simulink model "cds_simulink_file"  (R2020b)
settings: Solver=ode5  StartTime=0.0  StopTime=5  FixedStep=Ts  RelTol=1e-3
values from neighbouring files (symbols this model uses):
  D = (m2+mp/3)*9.81*[1;1;1;0]    [cds_main_bsmc_sigma.m]    (also in cds_model.m = ((m2+mp/3)*9.81)*[1;1;1;0]+external_force; cds_plant_sigma.m = ((m2+mp/3)*9.81+ef)*[1;1;1;0]; myIneqConFunction.m = ((m2+mp/3)*9.81)*[1;1;1;0]+external_force)
  PredictionHorizon = 5    [modelLyna_sm_withnoise (run first).m]
  Ts = 0.05    [modelLyna_sm_withnoise (run first).m]    (also in myIneqConFunction.m = data.Ts)
  u0 = [0;0;0;0]    [modelLyna_sm_withnoise (run first).m]
  x0 = [0*ones(3993,1); 0*ones(7,1)]    [cds_fuzzy_bsmc_sigma.m]    (also in cds_fuzzy_l_sigma.m; cds_main_bsmc_sigma.m = []; cds_plant_sigma.m = [0.45 0.7 0.5 0 0 0 0 0]; cds_setpoint_mpc.m = [])
undefined symbols (not defined in the file or in its folder): ref
libraries: mpclib x1
settings Model: Creator=Dell Precision  LastModifiedBy=Dell Precision
settings SFSimCC: CustomCodeUndefinedFunction=UseInterfaceOnly

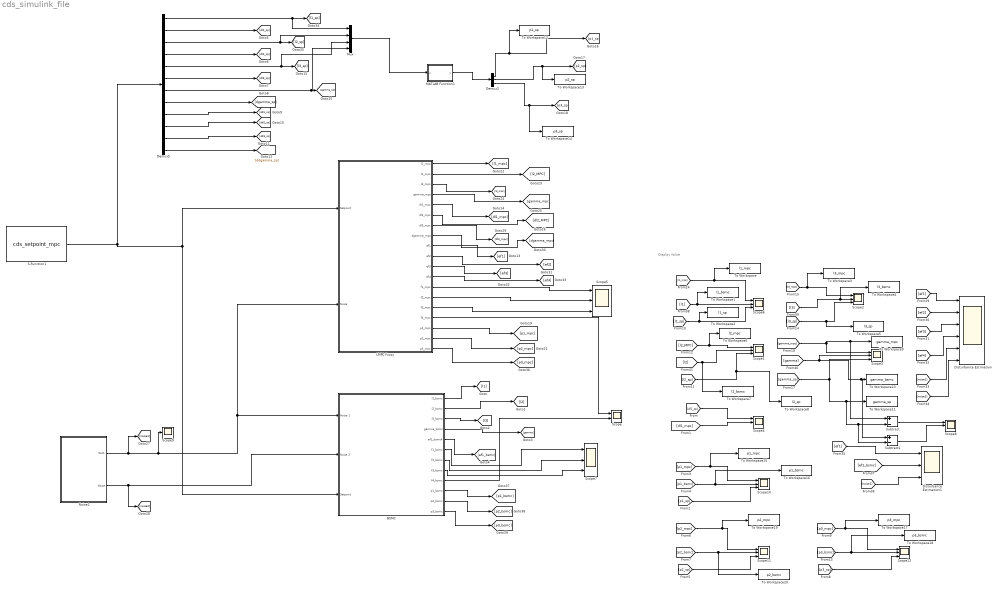
== system cds_simulink_file ==
  note: Display Value
  BSMC : Subsystem
  Demux2 : Demux  Outputs=3
  Demux5 : Demux  Outputs=12
  Disturbance Estimation : Scope  NumInputPorts=6
  Disturbance Estimation1 : Scope  NumInputPorts=3
  LMPC Fuzzy : Subsystem
  MATLAB Function1 : MATLAB Function  TreatAsAtomicUnit=on
  Mux : Mux
  Noise2 : Subsystem
  S-Function1 : S-Function  FunctionName=cds_setpoint_mpc  SFunctionDeploymentMode=off  EnableBusSupport=off
  Scope : Scope  NumInputPorts=2
  Scope{1..8,10..12} (11 alike) : Scope  NumInputPorts=3
  Scope9 : Scope
  Subtract : Sum  Inputs=+-
  Subtract1 : Sum  Inputs=+-
  To Workspace : ToWorkspace  VariableName=l1_mpc  SaveFormat=Timeseries  SampleTime=-1
  To Workspace1 : ToWorkspace  VariableName=l1_bsmc  SaveFormat=Timeseries  SampleTime=-1
  To Workspace10 : ToWorkspace  VariableName=gamma_bsmc  SaveFormat=Timeseries  SampleTime=-1
  To Workspace11 : ToWorkspace  VariableName=gamma_sp  SaveFormat=Timeseries  SampleTime=-1
  To Workspace12 : ToWorkspace  VariableName=p1_sp  SaveFormat=Timeseries  SampleTime=-1
  To Workspace13 : ToWorkspace  VariableName=p2_sp  SaveFormat=Timeseries  SampleTime=-1
  To Workspace14 : ToWorkspace  VariableName=p3_sp  SaveFormat=Timeseries  SampleTime=-1
  To Workspace15 : ToWorkspace  VariableName=p1_mpc  SaveFormat=Timeseries  SampleTime=-1
  To Workspace16 : ToWorkspace  VariableName=p1_bsmc  SaveFormat=Timeseries  SampleTime=-1
  To Workspace17 : ToWorkspace  VariableName=p3_mpc  SaveFormat=Timeseries  SampleTime=-1
  To Workspace18 : ToWorkspace  VariableName=p3_bsmc  SaveFormat=Timeseries  SampleTime=-1
  To Workspace19 : ToWorkspace  VariableName=p2_mpc  SaveFormat=Timeseries  SampleTime=-1
  To Workspace2 : ToWorkspace  VariableName=l1_sp  SaveFormat=Timeseries  SampleTime=-1
  To Workspace20 : ToWorkspace  VariableName=p2_bsmc  SaveFormat=Timeseries  SampleTime=-1
  To Workspace3 : ToWorkspace  VariableName=l3_mpc  SaveFormat=Timeseries  SampleTime=-1
  To Workspace4 : ToWorkspace  VariableName=l3_bsmc  SaveFormat=Timeseries  SampleTime=-1
  To Workspace5 : ToWorkspace  VariableName=l3_sp  SaveFormat=Timeseries  SampleTime=-1
  To Workspace6 : ToWorkspace  VariableName=l2_mpc  SaveFormat=Timeseries  SampleTime=-1
  To Workspace7 : ToWorkspace  VariableName=l2_bsmc  SaveFormat=Timeseries  SampleTime=-1
  To Workspace8 : ToWorkspace  VariableName=l2_sp  SaveFormat=Timeseries  SampleTime=-1
  To Workspace9 : ToWorkspace  VariableName=gamma_mpc  SaveFormat=Timeseries  SampleTime=-1
  wires:
  [l1_mpc] -> To Workspace/1, Scope6/1
  Noise2/2(Noise) -> BSMC/2(Noise 2), [noise2]
  [l3_sp] -> To Workspace5/1, Scope2/3
  [noise2] -> Disturbance Estimation/6
  [noise1] -> Disturbance Estimation/5
  [gamma_mpc] -> Subtract/1, To Workspace9/1, Scope3/1
  [l1_sp] -> To Workspace2/1, Scope6/3
  [l2_sp] -> To Workspace8/1, Scope1/3
  [ef2] -> Disturbance Estimation/2
  [ef1] -> Disturbance Estimation/1
  [ef3] -> Disturbance Estimation/3
  [l3_mpc] -> To Workspace3/1, Scope2/1
  [ef4] -> Disturbance Estimation/4
  Noise2/1(Out1) -> Scope9/1, LMPC Fuzzy/2(Noise), BSMC/1(Noise 1), [noise1]
  [gamma_sp] -> Subtract1/2, Subtract/2, To Workspace11/1, Scope3/3
  [ef1] -> Disturbance Estimation1/1
  [noise1] -> Disturbance Estimation1/3
  [ef1_bsmc] -> Disturbance Estimation1/2
  [l1] -> To Workspace1/1, Scope6/2
  [l3] -> To Workspace4/1, Scope2/2
  [gamma] -> Scope3/2, Subtract1/1, To Workspace10/1
  [l2] -> To Workspace7/1, Scope1/2
  LMPC Fuzzy/1(l1_mpc) -> [l1_mpc]
  LMPC Fuzzy/2(l2_mpc) -> [l2_MPC]
  LMPC Fuzzy/3(l3_mpc) -> [l3_mpc]
  LMPC Fuzzy/4(gamma_mpc) -> [gamma_mpc]
  LMPC Fuzzy/5(dl1_mpc) -> [dl1_mpc]
  LMPC Fuzzy/6(dl2_mpc) -> [dl2_MPC]
  LMPC Fuzzy/7(dl3_mpc) -> [dl3_mpc]
  LMPC Fuzzy/8(dgamma_mpc) -> [dgamma_mpc]
  LMPC Fuzzy/9(ef1) -> [ef1]
  LMPC Fuzzy/10(ef2) -> [ef2]
  LMPC Fuzzy/11(ef3) -> [ef3]
  LMPC Fuzzy/12(ef4) -> [ef4]
  [dl1_sp] -> Scope4/1
  [dl1_mpc] -> Scope4/2
  BSMC/1(l1_bsmc) -> [l1]
  BSMC/2(l2_bsmc) -> [l2]
  BSMC/3(l3_bsmc) -> [l3]
  BSMC/4(gamma_bsmc) -> [gamma]
  BSMC/5(ef1_bsmc4) -> [ef1_bsmc]
  Demux5/12 -> [ddgamma_sp]
  Demux5/8 -> [dgamma_sp]
  Demux5/9 -> [ddl1_sp]
  Demux5/5 -> Mux/3, [l3_sp]
  Demux5/4 -> [dl2_sp]
  S-Function1/1 -> Demux5/1, BSMC/3(Setpoint), LMPC Fuzzy/1(Setpoint)
  Demux5/2 -> [dl1_sp]
  Demux5/7 -> Mux/4, [gamma_sp]
  Demux5/10 -> [ddl2_sp]
  Demux5/3 -> Mux/2, [l2_sp]
  Demux5/1 -> Mux/1, [l1_sp]
  Demux5/11 -> [ddl3_sp]
  Demux5/6 -> [dl3_sp]
  [l2_MPC] -> To Workspace6/1, Scope1/1
  LMPC Fuzzy/13(f1_mpc) -> Scope5/1
  LMPC Fuzzy/14(f2_mpc) -> Scope5/2
  LMPC Fuzzy/15(f3_mpc) -> Scope5/3
  BSMC/6(f1_bsmc) -> Scope7/1
  BSMC/7(f2_bsmc) -> Scope7/2
  BSMC/8(f3_bsmc) -> Scope7/3
  LMPC Fuzzy/16(f4_mpc) -> Scope/1
  BSMC/9(f4_bsmc) -> Scope/2
  Subtract/1 -> Scope8/1
  Subtract1/1 -> Scope8/2
  Demux2/1 -> To Workspace12/1, [p1_sp]
  MATLAB Function1/1(y) -> Demux2/1
  Demux2/2 -> To Workspace13/1, [p2_sp]
  Demux2/3 -> To Workspace14/1, [p3_sp]
  Mux/1 -> MATLAB Function1/1(u)
  LMPC Fuzzy/17(p1_mpc) -> [p1_mpc]
  LMPC Fuzzy/18(p2_mpc) -> [p2_mpc]
  LMPC Fuzzy/19(p3_mpc) -> [p3_mpc]
  BSMC/10(p1_bsmc) -> [p1_bsmc]
  BSMC/11(p2_bsmc) -> [p2_bsmc]
  BSMC/12(p3_bsmc) -> [p3_bsmc]
  [p1_sp] -> Scope10/3
  [p2_mpc] -> To Workspace19/1, Scope11/1
  [p2_sp] -> Scope11/3
  [p2_bsmc] -> To Workspace20/1, Scope11/2
  [p3_bsmc] -> To Workspace18/1, Scope12/2
  [p3_sp] -> Scope12/3
  [p3_mpc] -> To Workspace17/1, Scope12/1
  [p1_mpc] -> To Workspace15/1, Scope10/1
  [p1_bsmc] -> To Workspace16/1, Scope10/2

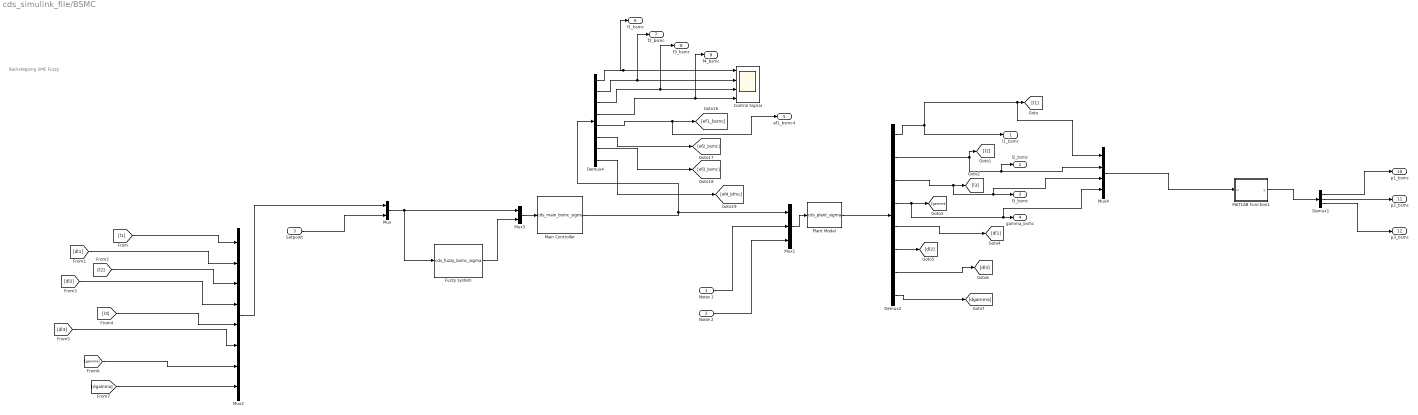
== system cds_simulink_file/BSMC ==
  note: Backstepping SMC Fuzzy
  Noise 1 : Inport
  Noise 2 : Inport  Port=2
  Setpoint : Inport  Port=3
  Control Signal : Scope  NumInputPorts=4
  Demux1 : Demux  Outputs=3
  Demux2 : Demux  Outputs=8
  Demux4 : Demux  Outputs=8
  Fuzzy system : S-Function  FunctionName=cds_fuzzy_bsmc_sigma  SFunctionDeploymentMode=off  EnableBusSupport=off
  MATLAB Function1 : MATLAB Function  TreatAsAtomicUnit=on
  Main Controller : S-Function  FunctionName=cds_main_bsmc_sigma  SFunctionDeploymentMode=off  EnableBusSupport=off
  Mux : Mux  Inputs=2
  Mux1 : Mux  Inputs=3
  Mux2 : Mux  Inputs=8
  Mux3 : Mux  Inputs=2
  Mux4 : Mux
  Plant Model : S-Function  FunctionName=cds_plant_sigma  SFunctionDeploymentMode=off  EnableBusSupport=off
  l1_bsmc : Outport
  l2_bsmc : Outport  Port=2
  l3_bsmc : Outport  Port=3
  gamma_bsmc : Outport  Port=4
  ef1_bsmc4 : Outport  Port=5
  f1_bsmc : Outport  Port=6
  f2_bsmc : Outport  Port=7
  f3_bsmc : Outport  Port=8
  f4_bsmc : Outport  Port=9
  p1_bsmc : Outport  Port=10
  p2_bsmc : Outport  Port=11
  p3_bsmc : Outport  Port=12
  wires:
  Demux4/4 -> f4_bsmc/1, Control Signal/4
  Mux/1 -> Mux3/1, Fuzzy system/1
  Fuzzy system/1 -> Mux3/2
  Demux2/6 -> [dl2]
  Main Controller/1 -> Demux4/1, Mux1/1
  Demux2/1 -> l1_bsmc/1, Mux4/1, [l1]
  [dl2] -> Mux2/4
  [gamma] -> Mux2/7
  Noise 2/1 -> Mux1/3
  [l3] -> Mux2/5
  [l2] -> Mux2/3
  Noise 1/1 -> Mux1/2
  [dgamma] -> Mux2/8
  [dl3] -> Mux2/6
  Demux4/6 -> [ef2_bsmc]
  Plant Model/1 -> Demux2/1
  Setpoint/1 -> Mux/2
  Demux4/8 -> [ef4_bfmc]
  Demux2/3 -> Mux4/3, l3_bsmc/1, [l3]
  Demux2/8 -> [dgamma]
  Demux4/5 -> ef1_bsmc4/1, [ef1_bsmc]
  Demux4/1 -> f1_bsmc/1, Control Signal/1
  Mux2/1 -> Mux/1
  Demux4/7 -> [ef3_bsmc]
  [dl1] -> Mux2/2
  [l1] -> Mux2/1
  Demux2/5 -> [dl1]
  Demux4/3 -> f3_bsmc/1, Control Signal/3
  Demux2/2 -> Mux4/2, l2_bsmc/1, [l2]
  Mux1/1 -> Plant Model/1
  Demux2/4 -> Mux4/4, gamma_bsmc/1, [gamma]
  Demux2/7 -> [dl3]
  Mux3/1 -> Main Controller/1
  Demux4/2 -> f2_bsmc/1, Control Signal/2
  Demux1/1 -> p1_bsmc/1
  MATLAB Function1/1(y) -> Demux1/1
  Demux1/2 -> p2_bsmc/1
  Demux1/3 -> p3_bsmc/1
  Mux4/1 -> MATLAB Function1/1(u)

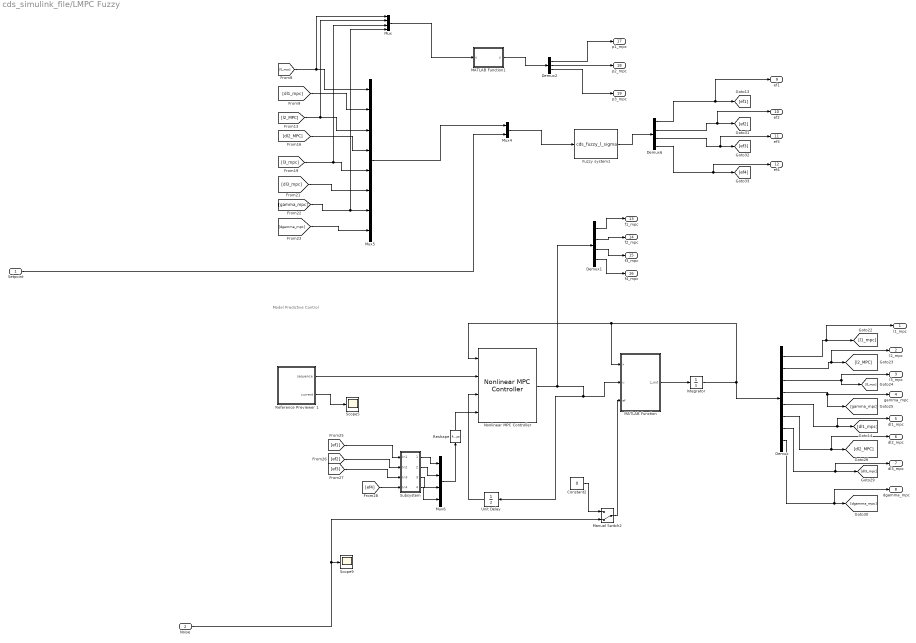
== system cds_simulink_file/LMPC Fuzzy ==
  note: Model Predictive Control
  Setpoint : Inport
  Noise : Inport  Port=2
  Constant2 : Constant  Value=0
  Demux : Demux  Outputs=8
  Demux1 : Demux
  Demux2 : Demux  Outputs=3
  Demux6 : Demux
  Fuzzy system1 : S-Function  FunctionName=cds_fuzzy_l_sigma  SFunctionDeploymentMode=off  EnableBusSupport=off
  Integrator : Integrator  InitialCondition=x0
  MATLAB Function : MATLAB Function  TreatAsAtomicUnit=on
  MATLAB Function1 : MATLAB Function  TreatAsAtomicUnit=on
  Manual Switch2 : ManualSwitch  CurrentSetting=0
  Mux : Mux
  Mux4 : Mux  Inputs=2
  Mux5 : Mux  Inputs=8
  Mux6 : Mux
  Nonlinear MPC Controller : mpclib/Nonlinear MPC Controller  SCDEnableBlockLinearizationSpecification=on  nlmpcobj=nlobj  UseObjectTs=on  UseMEX=off  md_enabled=on  mvtarget_enabled=off  param_enabled=off  cost_enabled=off  mvseq_enabled=off  stateseq_enabled=off  ovseq_enabled=off  slack_enabled=off  status_enabled=off  ov_min=off  ov_max=off  mv_min=off  mv_max=off  mvrate_min=off  mvrate_max=off  state_min=off  state_max=off  ov_weight=off  mv_weight=off  mvrate_weight=off  ecr_weight=off  nlp_initialize=off
  Reference Previewer 1 : Subsystem  mask{signal=ref, ts=Ts, steps=PredictionHorizon}
      mask prompts: signal "Signal name"; ts "Sampling time"; steps "Number of previewing steps"
      mask init:
      | ts = evalin('base',get_param(gcbh,'ts'));
      | signal = evalin('base',get_param(gcbh,'signal'));
      | steps = evalin('base',get_param(gcbh,'steps'));
      | data = mpc_previewer_maskinit(signal,ts);
      mask Display:
      | fprintf('Future\nsample\nextractor');
      | port_label('output', 1, 'seq')
      | port_label('output', 2, '@t')
  Reshape : Reshape  OutputDimensionality=Row vector (2-D)
  Scope5 : Scope
  Scope9 : Scope
  Subsystem : Subsystem
  Unit Delay : UnitDelay  InitialCondition=u0  SampleTime=-1  HasFrameUpgradeWarning=on
  l1_mpc : Outport
  l2_mpc : Outport  Port=2
  l3_mpc : Outport  Port=3
  gamma_mpc : Outport  Port=4
  dl1_mpc : Outport  Port=5
  dl2_mpc : Outport  Port=6
  dl3_mpc : Outport  Port=7
  dgamma_mpc : Outport  Port=8
  ef1 : Outport  Port=9
  ef2 : Outport  Port=10
  ef3 : Outport  Port=11
  ef4 : Outport  Port=12
  f1_mpc : Outport  Port=13
  f2_mpc : Outport  Port=14
  f3_mpc : Outport  Port=15
  f4_mpc : Outport  Port=16
  p1_mpc : Outport  Port=17
  p2_mpc : Outport  Port=18
  p3_mpc : Outport  Port=19
  wires:
  Manual Switch2/1 -> MATLAB Function/3(ef)
  Integrator/1 -> MATLAB Function/1(x), Nonlinear MPC Controller/1, Demux/1
  Demux/6 -> dl2_mpc/1, [dl2_MPC]
  Demux6/3 -> ef3/1, [ef3]
  [dl1_mpc] -> Mux5/2
  Demux/2 -> l2_mpc/1, [l2_MPC]
  MATLAB Function/1(z_out) -> Integrator/1
  Unit Delay/1 -> Nonlinear MPC Controller/3
  Demux6/4 -> ef4/1, [ef4]
  Demux6/2 -> ef2/1, [ef2]
  Reference Previewer 1/2(current) -> Scope5/1
  [dl2_MPC] -> Mux5/4
  [dl3_mpc] -> Mux5/6
  Mux6/1 -> Reshape/1
  Demux/5 -> dl1_mpc/1, [dl1_mpc]
  Noise/1 -> Manual Switch2/2, Scope9/1
  [ef4] -> Subsystem/4(In4)
  Demux/8 -> dgamma_mpc/1, [dgamma_mpc]
  Subsystem/1(Out1) -> Mux6/1
  Subsystem/3(Out3) -> Mux6/3
  [ef3] -> Subsystem/3(In3)
  Setpoint/1 -> Mux4/2
  [gamma_mpc] -> Mux/4, Mux5/7
  Fuzzy system1/1 -> Demux6/1
  Mux5/1 -> Mux4/1
  Reshape/1 -> Nonlinear MPC Controller/4
  Nonlinear MPC Controller/1 -> Demux1/1, MATLAB Function/2(u), Unit Delay/1
  Constant2/1 -> Manual Switch2/1
  Reference Previewer 1/1(sequence) -> Nonlinear MPC Controller/2
  Subsystem/4(Out4) -> Mux6/4
  Demux/3 -> l3_mpc/1, [l3_mpc]
  Subsystem/2(Out2) -> Mux6/2
  [l2_MPC] -> Mux/2, Mux5/3
  Demux/4 -> [gamma_mpc], gamma_mpc/1
  Demux/7 -> dl3_mpc/1, [dl3_mpc]
  [ef1] -> Subsystem/1(In1)
  [l1_mpc] -> Mux/1, Mux5/1
  Demux/1 -> l1_mpc/1, [l1_mpc]
  Mux4/1 -> Fuzzy system1/1
  [l3_mpc] -> Mux/3, Mux5/5
  [dgamma_mpc] -> Mux5/8
  [ef2] -> Subsystem/2(In2)
  Demux6/1 -> ef1/1, [ef1]
  Demux1/1 -> f1_mpc/1
  Demux1/2 -> f2_mpc/1
  Demux1/3 -> f3_mpc/1
  Demux1/4 -> f4_mpc/1
  Mux/1 -> MATLAB Function1/1(u)
  MATLAB Function1/1(y) -> Demux2/1
  Demux2/1 -> p1_mpc/1
  Demux2/2 -> p2_mpc/1
  Demux2/3 -> p3_mpc/1

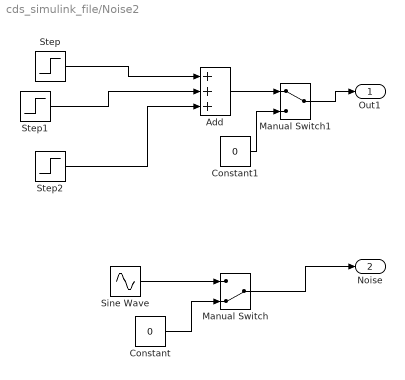
== system cds_simulink_file/Noise2 ==
  Add : Sum  Inputs=+++
  Constant : Constant  Value=0  SampleTime=-1
  Constant1 : Constant  Value=0  SampleTime=-1
  Manual Switch : ManualSwitch  CurrentSetting=0
  Manual Switch1 : ManualSwitch
  Sine Wave : Sin  Amplitude=25  Bias=25  Frequency=4  Phase=pi/2  SampleTime=0
  Step : Step  After=50  SampleTime=0
  Step1 : Step  Time=2  After=-80  SampleTime=0
  Step2 : Step  Time=4  After=60  SampleTime=0
  Out1 : Outport
  Noise : Outport  Port=2
  wires:
  Step/1 -> Add/1
  Step2/1 -> Add/3
  Step1/1 -> Add/2
  Sine Wave/1 -> Manual Switch/1
  Constant/1 -> Manual Switch/2
  Manual Switch/1 -> Noise/1
  Add/1 -> Manual Switch1/1
  Manual Switch1/1 -> Out1/1
  Constant1/1 -> Manual Switch1/2

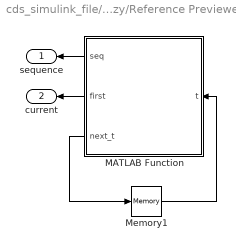
== system cds_simulink_file/LMPC Fuzzy/Reference Previewer 1 ==
  MATLAB Function : MATLAB Function  TreatAsAtomicUnit=on
  Memory1 : Memory  InheritSampleTime=on  LinearizeAsDelay=on
  sequence : Outport  VectorParamsAs1DForOutWhenUnconnected=off
  current : Outport  Port=2  VectorParamsAs1DForOutWhenUnconnected=off
  wires:
  MATLAB Function/1(seq) -> sequence/1
  MATLAB Function/2(first) -> current/1
  Memory1/1 -> MATLAB Function/1(t)
  MATLAB Function/3(next_t) -> Memory1/1

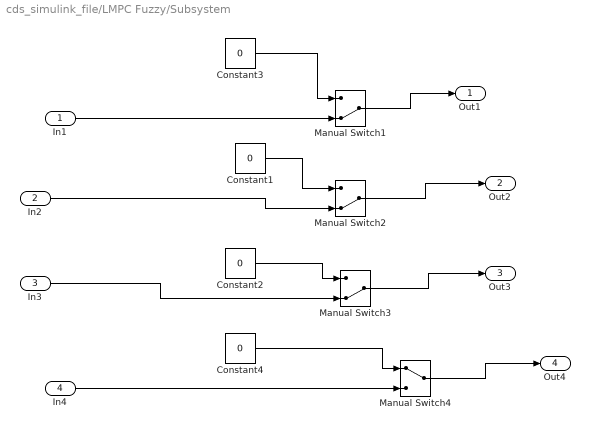
== system cds_simulink_file/LMPC Fuzzy/Subsystem ==
  In1 : Inport
  In2 : Inport  Port=2
  In3 : Inport  Port=3
  In4 : Inport  Port=4
  Constant{1..4} (4 alike) : Constant  Value=0
  Manual Switch1 : ManualSwitch  CurrentSetting=0
  Manual Switch2 : ManualSwitch  CurrentSetting=0
  Manual Switch3 : ManualSwitch  CurrentSetting=0
  Manual Switch4 : ManualSwitch
  Out1 : Outport
  Out2 : Outport  Port=2
  Out3 : Outport  Port=3
  Out4 : Outport  Port=4
  wires:
  Constant3/1 -> Manual Switch1/1
  Manual Switch1/1 -> Out1/1
  In1/1 -> Manual Switch1/2
  Manual Switch2/1 -> Out2/1
  Constant1/1 -> Manual Switch2/1
  Constant2/1 -> Manual Switch3/1
  Manual Switch3/1 -> Out3/1
  Manual Switch4/1 -> Out4/1
  Constant4/1 -> Manual Switch4/1
  In2/1 -> Manual Switch2/2
  In3/1 -> Manual Switch3/2
  In4/1 -> Manual Switch4/2

== matlab function cds_simulink_file/LMPC Fuzzy/MATLAB Function1 ==
  data: u input; y output
function y = cal_inv(u)

%% input

q = u(1:4);

l1 = q(1);
l2 = q(2);
l3 = q(3);
gamma = q(4);
a = 0.5;
az = 0.05;

A1 = [a*sin(pi/6) a*cos(pi/6) 0]';
A2 = [-a 0 0]';
A3 = [a*sin(pi/6) -a*cos(pi/6) 0]';


B1 = [a*sin(pi/6) a*cos(pi/6) 0]';
B2 = [-a 0 0]';
B3 = [a*sin(pi/6) -a*cos(pi/6) 0]';



X = [150;0;0];

for i = 1:100

    Pz = X(1);    
    alpha = X(2);
    beta = X(3);

Rp = [cos(beta)*cos(gamma) cos(gamma)*sin(alpha)*sin(beta)-cos(alpha)*sin(gamma) sin(alpha)*sin(gamma)+cos(alpha)*cos(gamma)*sin(beta);
      cos(beta)*sin(gamma) cos(alpha)*cos(gamma)+sin(alpha)*sin(beta)*sin(gamma) cos(alpha)*sin(beta)*sin(gamma)-cos(gamma)*sin(alpha);
      -sin(beta)                    cos(beta)*sin(alpha)                                        cos(alpha)*cos(beta)                   ];
Ra = [cos(gamma) -sin(gamma) 0;
      sin(gamma) cos(gamma)  0; 
           0         0       1];
       


Oa = [0 0 az]';
P  = [0 0 Pz]';

f1 = (Rp*B1 + P - Ra*A1 - Oa)'*(Rp*B1 + P - Ra*A1 - Oa) - l1^2  ;
f2 = (Rp*B2 + P - Ra*A2 - Oa)'*(Rp*B2 + P - Ra*A2 - Oa) - l2^2  ;
f3 = (Rp*B3 + P - Ra*A3 - Oa)'*(Rp*B3 + P - Ra*A3 - Oa) - l3^2  ;

df1z = Pz - az + conj(Pz) - conj(az) - (a*sin(conj(beta)))/2 - (conj(a)*sin(beta))/2 + (3^(1/2)*conj(a)*cos(beta)*sin(alpha))/2 + (3^(1/2)*a*cos(conj(beta))*sin(conj(alpha)))/2;
 
 
df1_alpha = (3^(1/2)*a*(cos(conj(gamma))*sin(conj(alpha)) - cos(conj(alpha))*sin(conj(beta))*sin(conj(gamma)))*((conj(a)*sin(gamma))/2 + (3^(1/2)*conj(a)*cos(gamma))/2 - (conj(a)*cos(beta)*cos(gamma))/2 - (3^(1/2)*conj(a)*(cos(alpha)*cos(gamma) + sin(alpha)*sin(beta)*sin(gamma)))/2))/2 - (3^(1/2)*a*(sin(conj(alpha))*sin(conj(gamma)) + cos(conj(alpha))*cos(conj(gamma))*sin(conj(beta)))*((conj(a)*cos(gamma))/2 - (3^(1/2)*conj(a)*sin(gamma))/2 - (conj(a)*cos(beta)*cos(gamma))/2 + (3^(1/2)*conj(a)*(cos(alpha)*sin(gamma) - cos(gamma)*sin(alpha)*sin(beta)))/2))/2 - (3^(1/2)*conj(a)*(sin(alpha)*sin(gamma) + cos(alpha)*cos(gamma)*sin(beta))*((a*cos(conj(gamma)))/2 - (a*cos(conj(beta))*cos(conj(gamma)))/2 + (3^(1/2)*a*(cos(conj(alpha))*sin(conj(gamma)) - cos(conj(gamma))*sin(conj(alpha))*sin(conj(beta))))/2 - (3^(1/2)*a*sin(conj(gamma)))/2))/2 + (3^(1/2)*conj(a)*(cos(gamma)*sin(alpha) - cos(alpha)*sin(beta)*sin(gamma))*((a*sin(conj(gamma)))/2 - (a*cos(conj(beta))*cos(conj(gamma)))/2 - (3^(1/2)*a*(cos(conj(alpha))*cos(conj(gamma)) + sin(conj(alpha))*sin(conj(beta))*sin(conj(gamma))))/2 + (3^(1/2)*a*cos(conj(gamma)))/2))/2 + (3^(1/2)*a*cos(conj(alpha))*cos(conj(beta))*(conj(Pz) - conj(az) - (conj(a)*sin(beta))/2 + (3^(1/2)*conj(a)*cos(beta)*sin(alpha))/2))/2 + (3^(1/2)*conj(a)*cos(alpha)*cos(beta)*(Pz - az - (a*sin(conj(beta)))/2 + (3^(1/2)*a*cos(conj(beta))*sin(conj(alpha)))/2))/2;
 
 
df1_beta = ((conj(a)*cos(gamma)*sin(beta))/2 - (3^(1/2)*conj(a)*cos(beta)*cos(gamma)*sin(alpha))/2)*((a*cos(conj(gamma)))/2 - (a*cos(conj(beta))*cos(conj(gamma)))/2 + (3^(1/2)*a*(cos(conj(alpha))*sin(conj(gamma)) - cos(conj(gamma))*sin(conj(alpha))*sin(conj(beta))))/2 - (3^(1/2)*a*sin(conj(gamma)))/2) + ((conj(a)*cos(gamma)*sin(beta))/2 - (3^(1/2)*conj(a)*cos(beta)*sin(alpha)*sin(gamma))/2)*((a*sin(conj(gamma)))/2 - (a*cos(conj(beta))*cos(conj(gamma)))/2 - (3^(1/2)*a*(cos(conj(alpha))*cos(conj(gamma)) + sin(conj(alpha))*sin(conj(beta))*sin(conj(gamma))))/2 + (3^(1/2)*a*cos(conj(gamma)))/2) - ((a*cos(conj(beta)))/2 + (3^(1/2)*a*sin(conj(alpha))*sin(conj(beta)))/2)*(conj(Pz) - conj(az) - (conj(a)*sin(beta))/2 + (3^(1/2)*conj(a)*cos(beta)*sin(alpha))/2) + ((a*cos(conj(gamma))*sin(conj(beta)))/2 - (3^(1/2)*a*cos(conj(beta))*cos(conj(gamma))*sin(conj(alpha)))/2)*((conj(a)*cos(gamma))/2 - (3^(1/2)*conj(a)*sin(gamma))/2 - (conj(a)*cos(beta)*cos(gamma))/2 + (3^(1/2)*conj(a)*(cos(alpha)*sin(gamma) - cos(gamma)*sin(alpha)*sin(beta)))/2) + ((a*cos(conj(gamma))*sin(conj(beta)))/2 - (3^(1/2)*a*cos(conj(beta))*sin(conj(alpha))*sin(conj(gamma)))/2)*((conj(a)*sin(gamma))/2 + (3^(1/2)*conj(a)*cos(gamma))/2 - (conj(a)*cos(beta)*cos(gamma))/2 - (3^(1/2)*conj(a)*(cos(alpha)*cos(gamma) + sin(alpha)*sin(beta)*sin(gamma)))/2) - ((conj(a)*cos(beta))/2 + (3^(1/2)*conj(a)*sin(alpha)*sin(beta))/2)*(Pz - az - (a*sin(conj(beta)))/2 + (3^(1/2)*a*cos(conj(beta))*sin(conj(alpha)))/2);
 
 
df2z = Pz - az + conj(Pz) - conj(az) + a*sin(conj(beta)) + conj(a)*sin(beta);
 
 
df2_alpha = 0;
 
 
df2_beta = a*cos(conj(beta))*(conj(Pz) - conj(az) + conj(a)*sin(beta)) + conj(a)*cos(beta)*(Pz - az + a*sin(conj(beta))) + a*cos(conj(gamma))*sin(conj(beta))*(conj(a)*cos(gamma) - conj(a)*cos(beta)*cos(gamma)) + conj(a)*cos(gamma)*sin(beta)*(a*cos(conj(gamma)) - a*cos(conj(beta))*cos(conj(gamma))) + a*cos(conj(gamma))*sin(conj(beta))*(conj(a)*sin(gamma) - conj(a)*cos(beta)*cos(gamma)) + conj(a)*cos(gamma)*sin(beta)*(a*sin(conj(gamma)) - a*cos(conj(beta))*cos(conj(gamma)));
 
 
df3z = Pz - az + conj(Pz) - conj(az) - (a*sin(conj(beta)))/2 - (conj(a)*sin(beta))/2 - (3^(1/2)*conj(a)*cos(beta)*sin(alpha))/2 - (3^(1/2)*a*cos(conj(beta))*sin(conj(alpha)))/2;
 
 
df3_alpha = (3^(1/2)*a*(sin(conj(alpha))*sin(conj(gamma)) + cos(conj(alpha))*cos(conj(gamma))*sin(conj(beta)))*((conj(a)*cos(gamma))/2 + (3^(1/2)*conj(a)*sin(gamma))/2 - (conj(a)*cos(beta)*cos(gamma))/2 - (3^(1/2)*conj(a)*(cos(alpha)*sin(gamma) - cos(gamma)*sin(alpha)*sin(beta)))/2))/2 - (3^(1/2)*a*(cos(conj(gamma))*sin(conj(alpha)) - cos(conj(alpha))*sin(conj(beta))*sin(conj(gamma)))*((conj(a)*sin(gamma))/2 - (3^(1/2)*conj(a)*cos(gamma))/2 - (conj(a)*cos(beta)*cos(gamma))/2 + (3^(1/2)*conj(a)*(cos(alpha)*cos(gamma) + sin(alpha)*sin(beta)*sin(gamma)))/2))/2 + (3^(1/2)*conj(a)*(sin(alpha)*sin(gamma) + cos(alpha)*cos(gamma)*sin(beta))*((a*cos(conj(gamma)))/2 - (a*cos(conj(beta))*cos(conj(gamma)))/2 - (3^(1/2)*a*(cos(conj(alpha))*sin(conj(gamma)) - cos(conj(gamma))*sin(conj(alpha))*sin(conj(beta))))/2 + (3^(1/2)*a*sin(conj(gamma)))/2))/2 - (3^(1/2)*conj(a)*(cos(gamma)*sin(alpha) - cos(alpha)*sin(beta)*sin(gamma))*((a*sin(conj(gamma)))/2 - (a*cos(conj(beta))*cos(conj(gamma)))/2 + (3^(1/2)*a*(cos(conj(alpha))*cos(conj(gamma)) + sin(conj(alpha))*sin(conj(beta))*sin(conj(gamma))))/2 - (3^(1/2)*a*cos(conj(gamma)))/2))/2 + (3^(1/2)*a*cos(conj(alpha))*cos(conj(beta))*(conj(az) - conj(Pz) + (conj(a)*sin(beta))/2 + (3^(1/2)*conj(a)*cos(beta)*sin(alpha))/2))/2 + (3^(1/2)*conj(a)*cos(alpha)*cos(beta)*(az - Pz + (a*sin(conj(beta)))/2 + (3^(1/2)*a*cos(conj(beta))*sin(conj(alpha)))/2))/2;
 
 
df3_beta = ((conj(a)*cos(gamma)*sin(beta))/2 + (3^(1/2)*conj(a)*cos(beta)*cos(gamma)*sin(alpha))/2)*((a*cos(conj(gamma)))/2 - (a*cos(conj(beta))*cos(conj(gamma)))/2 - (3^(1/2)*a*(cos(conj(alpha))*sin(conj(gamma)) - cos(conj(gamma))*sin(conj(alpha))*sin(conj(beta))))/2 + (3^(1/2)*a*sin(conj(gamma)))/2) + ((conj(a)*cos(gamma)*sin(beta))/2 + (3^(1/2)*conj(a)*cos(beta)*sin(alpha)*sin(gamma))/2)*((a*sin(conj(gamma)))/2 - (a*cos(conj(beta))*cos(conj(gamma)))/2 + (3^(1/2)*a*(cos(conj(alpha))*cos(conj(gamma)) + sin(conj(alpha))*sin(conj(beta))*sin(conj(gamma))))/2 - (3^(1/2)*a*cos(conj(gamma)))/2) + ((a*cos(conj(beta)))/2 - (3^(1/2)*a*sin(conj(alpha))*sin(conj(beta)))/2)*(conj(az) - conj(Pz) + (conj(a)*sin(beta))/2 + (3^(1/2)*conj(a)*cos(beta)*sin(alpha))/2) + ((a*cos(conj(gamma))*sin(conj(beta)))/2 + (3^(1/2)*a*cos(conj(beta))*cos(conj(gamma))*sin(conj(alpha)))/2)*((conj(a)*cos(gamma))/2 + (3^(1/2)*conj(a)*sin(gamma))/2 - (conj(a)*cos(beta)*cos(gamma))/2 - (3^(1/2)*conj(a)*(cos(alpha)*sin(gamma) - cos(gamma)*sin(alpha)*sin(beta)))/2) + ((a*cos(conj(gamma))*sin(conj(beta)))/2 + (3^(1/2)*a*cos(conj(beta))*sin(conj(alpha))*sin(conj(gamma)))/2)*((conj(a)*sin(gamma))/2 - (3^(1/2)*conj(a)*cos(gamma))/2 - (conj(a)*cos(beta)*cos(gamma))/2 + (3^(1/2)*conj(a)*(cos(alpha)*cos(gamma) + sin(alpha)*sin(beta)*sin(gamma)))/2) + ((conj(a)*cos(beta))/2 - (3^(1/2)*conj(a)*sin(alpha)*sin(beta))/2)*(az - Pz + (a*sin(conj(beta)))/2 + (3^(1/2)*a*cos(conj(beta))*sin(conj(alpha)))/2);

f = [f1 f2 f3]';

df = [df1z df1_alpha df1_beta;
      df2z df2_alpha df2_beta;   
      df3z df3_alpha df3_beta];

  
X = X - (df^(-1))*f;

end
 
X(1) = abs(X(1));
y = X;

end

== matlab function cds_simulink_file/LMPC Fuzzy/MATLAB Function ==
  data: x input; u input; z_out output; ef input
function z_out  = cds_model_sm(x,u, ef)

a = 0.5 ;                            % Some static parameters
mp = 15; m1 =0.5; m2 = 3; mdc =3; Ipy = 1; Ipx = 1; Igamma = 1;
m11 = m2 + mdc + mp/9 + Ipy/(4*a^2); m21 = mp/9;
m22 = m2+mdc+mp/9+ Ipx/(12*a^2); m33 = m2 +mdc +mp/9; m44 = Igamma;
M = [m11 m21 m21 0; m21 m22 m21 0; m21 m21 m33 0; 0 0 0 m44];
invM = inv(M);
c1 = 15*Ipy/(4*a^4) ; c2 = 5*Ipx/(12*a^4);
D = ((m2+mp/3)*9.81)*[1;1;1;0]+ ef*[1;1;1;0];

dl1 = x(5);
dl2 = x(6);
dl3 = x(7);
dgamma = x(8);
ddl1 =invM(1,1)*(u(1)-D(1)-c1*dl1*dl1)+invM(1,2)*(u(2) - D(2)-c2*dl2*dl2)+invM(1,3)*(u(3)-D(3))+invM(1,4)*(u(4)-D(4));
ddl2 =invM(2,1)*(u(1)-D(1)-c1*dl1*dl1)+invM(2,2)*(u(2) - D(2)-c2*dl2*dl2)+invM(2,3)*(u(3)-D(3))+invM(2,4)*(u(4)-D(4));
ddl3 =invM(3,1)*(u(1)-D(1)-c1*dl1*dl1)+invM(3,2)*(u(2) - D(2)-c2*dl2*dl2)+invM(3,3)*(u(3)-D(3))+invM(3,4)*(u(4)-D(4));
ddgamma =invM(4,4)*(u(4)-D(4));

z_out = [dl1;dl2;dl3;dgamma;ddl1;ddl2;ddl3;ddgamma];
end

== matlab function cds_simulink_file/LMPC Fuzzy/Reference Previewer 1/MATLAB Function ==
  settings: updateMethod=DISCRETE  sampleTime=ts
  data: data parameter; seq output; steps parameter; t input; first output; next_t output
function [seq,first,next_t] = fcn(data,steps,t)
%#codegen
[seq,first,next_t] = mpcblock_preview('ref',data,steps,t);

== matlab function cds_simulink_file/BSMC/MATLAB Function1 ==
  data: u input; y output
function y = cal_inv(u)

%% input

q = u(1:4);

l1 = q(1);
l2 = q(2);
l3 = q(3);
gamma = q(4);
a = 0.5;
az = 0.05;

A1 = [a*sin(pi/6) a*cos(pi/6) 0]';
A2 = [-a 0 0]';
A3 = [a*sin(pi/6) -a*cos(pi/6) 0]';


B1 = [a*sin(pi/6) a*cos(pi/6) 0]';
B2 = [-a 0 0]';
B3 = [a*sin(pi/6) -a*cos(pi/6) 0]';



X = [150;0;0];

for i = 1:100

    Pz = X(1);    
    alpha = X(2);
    beta = X(3);

Rp = [cos(beta)*cos(gamma) cos(gamma)*sin(alpha)*sin(beta)-cos(alpha)*sin(gamma) sin(alpha)*sin(gamma)+cos(alpha)*cos(gamma)*sin(beta);
      cos(beta)*sin(gamma) cos(alpha)*cos(gamma)+sin(alpha)*sin(beta)*sin(gamma) cos(alpha)*sin(beta)*sin(gamma)-cos(gamma)*sin(alpha);
      -sin(beta)                    cos(beta)*sin(alpha)                                        cos(alpha)*cos(beta)                   ];
Ra = [cos(gamma) -sin(gamma) 0;
      sin(gamma) cos(gamma)  0; 
           0         0       1];
       


Oa = [0 0 az]';
P  = [0 0 Pz]';

f1 = (Rp*B1 + P - Ra*A1 - Oa)'*(Rp*B1 + P - Ra*A1 - Oa) - l1^2  ;
f2 = (Rp*B2 + P - Ra*A2 - Oa)'*(Rp*B2 + P - Ra*A2 - Oa) - l2^2  ;
f3 = (Rp*B3 + P - Ra*A3 - Oa)'*(Rp*B3 + P - Ra*A3 - Oa) - l3^2  ;

df1z = Pz - az + conj(Pz) - conj(az) - (a*sin(conj(beta)))/2 - (conj(a)*sin(beta))/2 + (3^(1/2)*conj(a)*cos(beta)*sin(alpha))/2 + (3^(1/2)*a*cos(conj(beta))*sin(conj(alpha)))/2;
 
 
df1_alpha = (3^(1/2)*a*(cos(conj(gamma))*sin(conj(alpha)) - cos(conj(alpha))*sin(conj(beta))*sin(conj(gamma)))*((conj(a)*sin(gamma))/2 + (3^(1/2)*conj(a)*cos(gamma))/2 - (conj(a)*cos(beta)*cos(gamma))/2 - (3^(1/2)*conj(a)*(cos(alpha)*cos(gamma) + sin(alpha)*sin(beta)*sin(gamma)))/2))/2 - (3^(1/2)*a*(sin(conj(alpha))*sin(conj(gamma)) + cos(conj(alpha))*cos(conj(gamma))*sin(conj(beta)))*((conj(a)*cos(gamma))/2 - (3^(1/2)*conj(a)*sin(gamma))/2 - (conj(a)*cos(beta)*cos(gamma))/2 + (3^(1/2)*conj(a)*(cos(alpha)*sin(gamma) - cos(gamma)*sin(alpha)*sin(beta)))/2))/2 - (3^(1/2)*conj(a)*(sin(alpha)*sin(gamma) + cos(alpha)*cos(gamma)*sin(beta))*((a*cos(conj(gamma)))/2 - (a*cos(conj(beta))*cos(conj(gamma)))/2 + (3^(1/2)*a*(cos(conj(alpha))*sin(conj(gamma)) - cos(conj(gamma))*sin(conj(alpha))*sin(conj(beta))))/2 - (3^(1/2)*a*sin(conj(gamma)))/2))/2 + (3^(1/2)*conj(a)*(cos(gamma)*sin(alpha) - cos(alpha)*sin(beta)*sin(gamma))*((a*sin(conj(gamma)))/2 - (a*cos(conj(beta))*cos(conj(gamma)))/2 - (3^(1/2)*a*(cos(conj(alpha))*cos(conj(gamma)) + sin(conj(alpha))*sin(conj(beta))*sin(conj(gamma))))/2 + (3^(1/2)*a*cos(conj(gamma)))/2))/2 + (3^(1/2)*a*cos(conj(alpha))*cos(conj(beta))*(conj(Pz) - conj(az) - (conj(a)*sin(beta))/2 + (3^(1/2)*conj(a)*cos(beta)*sin(alpha))/2))/2 + (3^(1/2)*conj(a)*cos(alpha)*cos(beta)*(Pz - az - (a*sin(conj(beta)))/2 + (3^(1/2)*a*cos(conj(beta))*sin(conj(alpha)))/2))/2;
 
 
df1_beta = ((conj(a)*cos(gamma)*sin(beta))/2 - (3^(1/2)*conj(a)*cos(beta)*cos(gamma)*sin(alpha))/2)*((a*cos(conj(gamma)))/2 - (a*cos(conj(beta))*cos(conj(gamma)))/2 + (3^(1/2)*a*(cos(conj(alpha))*sin(conj(gamma)) - cos(conj(gamma))*sin(conj(alpha))*sin(conj(beta))))/2 - (3^(1/2)*a*sin(conj(gamma)))/2) + ((conj(a)*cos(gamma)*sin(beta))/2 - (3^(1/2)*conj(a)*cos(beta)*sin(alpha)*sin(gamma))/2)*((a*sin(conj(gamma)))/2 - (a*cos(conj(beta))*cos(conj(gamma)))/2 - (3^(1/2)*a*(cos(conj(alpha))*cos(conj(gamma)) + sin(conj(alpha))*sin(conj(beta))*sin(conj(gamma))))/2 + (3^(1/2)*a*cos(conj(gamma)))/2) - ((a*cos(conj(beta)))/2 + (3^(1/2)*a*sin(conj(alpha))*sin(conj(beta)))/2)*(conj(Pz) - conj(az) - (conj(a)*sin(beta))/2 + (3^(1/2)*conj(a)*cos(beta)*sin(alpha))/2) + ((a*cos(conj(gamma))*sin(conj(beta)))/2 - (3^(1/2)*a*cos(conj(beta))*cos(conj(gamma))*sin(conj(alpha)))/2)*((conj(a)*cos(gamma))/2 - (3^(1/2)*conj(a)*sin(gamma))/2 - (conj(a)*cos(beta)*cos(gamma))/2 + (3^(1/2)*conj(a)*(cos(alpha)*sin(gamma) - cos(gamma)*sin(alpha)*sin(beta)))/2) + ((a*cos(conj(gamma))*sin(conj(beta)))/2 - (3^(1/2)*a*cos(conj(beta))*sin(conj(alpha))*sin(conj(gamma)))/2)*((conj(a)*sin(gamma))/2 + (3^(1/2)*conj(a)*cos(gamma))/2 - (conj(a)*cos(beta)*cos(gamma))/2 - (3^(1/2)*conj(a)*(cos(alpha)*cos(gamma) + sin(alpha)*sin(beta)*sin(gamma)))/2) - ((conj(a)*cos(beta))/2 + (3^(1/2)*conj(a)*sin(alpha)*sin(beta))/2)*(Pz - az - (a*sin(conj(beta)))/2 + (3^(1/2)*a*cos(conj(beta))*sin(conj(alpha)))/2);
 
 
df2z = Pz - az + conj(Pz) - conj(az) + a*sin(conj(beta)) + conj(a)*sin(beta);
 
 
df2_alpha = 0;
 
 
df2_beta = a*cos(conj(beta))*(conj(Pz) - conj(az) + conj(a)*sin(beta)) + conj(a)*cos(beta)*(Pz - az + a*sin(conj(beta))) + a*cos(conj(gamma))*sin(conj(beta))*(conj(a)*cos(gamma) - conj(a)*cos(beta)*cos(gamma)) + conj(a)*cos(gamma)*sin(beta)*(a*cos(conj(gamma)) - a*cos(conj(beta))*cos(conj(gamma))) + a*cos(conj(gamma))*sin(conj(beta))*(conj(a)*sin(gamma) - conj(a)*cos(beta)*cos(gamma)) + conj(a)*cos(gamma)*sin(beta)*(a*sin(conj(gamma)) - a*cos(conj(beta))*cos(conj(gamma)));
 
 
df3z = Pz - az + conj(Pz) - conj(az) - (a*sin(conj(beta)))/2 - (conj(a)*sin(beta))/2 - (3^(1/2)*conj(a)*cos(beta)*sin(alpha))/2 - (3^(1/2)*a*cos(conj(beta))*sin(conj(alpha)))/2;
 
 
df3_alpha = (3^(1/2)*a*(sin(conj(alpha))*sin(conj(gamma)) + cos(conj(alpha))*cos(conj(gamma))*sin(conj(beta)))*((conj(a)*cos(gamma))/2 + (3^(1/2)*conj(a)*sin(gamma))/2 - (conj(a)*cos(beta)*cos(gamma))/2 - (3^(1/2)*conj(a)*(cos(alpha)*sin(gamma) - cos(gamma)*sin(alpha)*sin(beta)))/2))/2 - (3^(1/2)*a*(cos(conj(gamma))*sin(conj(alpha)) - cos(conj(alpha))*sin(conj(beta))*sin(conj(gamma)))*((conj(a)*sin(gamma))/2 - (3^(1/2)*conj(a)*cos(gamma))/2 - (conj(a)*cos(beta)*cos(gamma))/2 + (3^(1/2)*conj(a)*(cos(alpha)*cos(gamma) + sin(alpha)*sin(beta)*sin(gamma)))/2))/2 + (3^(1/2)*conj(a)*(sin(alpha)*sin(gamma) + cos(alpha)*cos(gamma)*sin(beta))*((a*cos(conj(gamma)))/2 - (a*cos(conj(beta))*cos(conj(gamma)))/2 - (3^(1/2)*a*(cos(conj(alpha))*sin(conj(gamma)) - cos(conj(gamma))*sin(conj(alpha))*sin(conj(beta))))/2 + (3^(1/2)*a*sin(conj(gamma)))/2))/2 - (3^(1/2)*conj(a)*(cos(gamma)*sin(alpha) - cos(alpha)*sin(beta)*sin(gamma))*((a*sin(conj(gamma)))/2 - (a*cos(conj(beta))*cos(conj(gamma)))/2 + (3^(1/2)*a*(cos(conj(alpha))*cos(conj(gamma)) + sin(conj(alpha))*sin(conj(beta))*sin(conj(gamma))))/2 - (3^(1/2)*a*cos(conj(gamma)))/2))/2 + (3^(1/2)*a*cos(conj(alpha))*cos(conj(beta))*(conj(az) - conj(Pz) + (conj(a)*sin(beta))/2 + (3^(1/2)*conj(a)*cos(beta)*sin(alpha))/2))/2 + (3^(1/2)*conj(a)*cos(alpha)*cos(beta)*(az - Pz + (a*sin(conj(beta)))/2 + (3^(1/2)*a*cos(conj(beta))*sin(conj(alpha)))/2))/2;
 
 
df3_beta = ((conj(a)*cos(gamma)*sin(beta))/2 + (3^(1/2)*conj(a)*cos(beta)*cos(gamma)*sin(alpha))/2)*((a*cos(conj(gamma)))/2 - (a*cos(conj(beta))*cos(conj(gamma)))/2 - (3^(1/2)*a*(cos(conj(alpha))*sin(conj(gamma)) - cos(conj(gamma))*sin(conj(alpha))*sin(conj(beta))))/2 + (3^(1/2)*a*sin(conj(gamma)))/2) + ((conj(a)*cos(gamma)*sin(beta))/2 + (3^(1/2)*conj(a)*cos(beta)*sin(alpha)*sin(gamma))/2)*((a*sin(conj(gamma)))/2 - (a*cos(conj(beta))*cos(conj(gamma)))/2 + (3^(1/2)*a*(cos(conj(alpha))*cos(conj(gamma)) + sin(conj(alpha))*sin(conj(beta))*sin(conj(gamma))))/2 - (3^(1/2)*a*cos(conj(gamma)))/2) + ((a*cos(conj(beta)))/2 - (3^(1/2)*a*sin(conj(alpha))*sin(conj(beta)))/2)*(conj(az) - conj(Pz) + (conj(a)*sin(beta))/2 + (3^(1/2)*conj(a)*cos(beta)*sin(alpha))/2) + ((a*cos(conj(gamma))*sin(conj(beta)))/2 + (3^(1/2)*a*cos(conj(beta))*cos(conj(gamma))*sin(conj(alpha)))/2)*((conj(a)*cos(gamma))/2 + (3^(1/2)*conj(a)*sin(gamma))/2 - (conj(a)*cos(beta)*cos(gamma))/2 - (3^(1/2)*conj(a)*(cos(alpha)*sin(gamma) - cos(gamma)*sin(alpha)*sin(beta)))/2) + ((a*cos(conj(gamma))*sin(conj(beta)))/2 + (3^(1/2)*a*cos(conj(beta))*sin(conj(alpha))*sin(conj(gamma)))/2)*((conj(a)*sin(gamma))/2 - (3^(1/2)*conj(a)*cos(gamma))/2 - (conj(a)*cos(beta)*cos(gamma))/2 + (3^(1/2)*conj(a)*(cos(alpha)*cos(gamma) + sin(alpha)*sin(beta)*sin(gamma)))/2) + ((conj(a)*cos(beta))/2 - (3^(1/2)*conj(a)*sin(alpha)*sin(beta))/2)*(az - Pz + (a*sin(conj(beta)))/2 + (3^(1/2)*a*cos(conj(beta))*sin(conj(alpha)))/2);

f = [f1 f2 f3]';

df = [df1z df1_alpha df1_beta;
      df2z df2_alpha df2_beta;   
      df3z df3_alpha df3_beta];

  
X = X - (df^(-1))*f;

end
 
X(1) = abs(X(1));
y = X;

end

== matlab function cds_simulink_file/MATLAB Function1 ==
  data: u input; y output
function y = cal_inv(u)

%% input

q = u(1:4);

l1 = q(1);
l2 = q(2);
l3 = q(3);
gamma = q(4);
a = 0.5;
az = 0.05;

A1 = [a*sin(pi/6) a*cos(pi/6) 0]';
A2 = [-a 0 0]';
A3 = [a*sin(pi/6) -a*cos(pi/6) 0]';


B1 = [a*sin(pi/6) a*cos(pi/6) 0]';
B2 = [-a 0 0]';
B3 = [a*sin(pi/6) -a*cos(pi/6) 0]';



X = [150;0;0];

for i = 1:100

    Pz = X(1);    
    alpha = X(2);
    beta = X(3);

Rp = [cos(beta)*cos(gamma) cos(gamma)*sin(alpha)*sin(beta)-cos(alpha)*sin(gamma) sin(alpha)*sin(gamma)+cos(alpha)*cos(gamma)*sin(beta);
      cos(beta)*sin(gamma) cos(alpha)*cos(gamma)+sin(alpha)*sin(beta)*sin(gamma) cos(alpha)*sin(beta)*sin(gamma)-cos(gamma)*sin(alpha);
      -sin(beta)                    cos(beta)*sin(alpha)                                        cos(alpha)*cos(beta)                   ];
Ra = [cos(gamma) -sin(gamma) 0;
      sin(gamma) cos(gamma)  0; 
           0         0       1];
       


Oa = [0 0 az]';
P  = [0 0 Pz]';

f1 = (Rp*B1 + P - Ra*A1 - Oa)'*(Rp*B1 + P - Ra*A1 - Oa) - l1^2  ;
f2 = (Rp*B2 + P - Ra*A2 - Oa)'*(Rp*B2 + P - Ra*A2 - Oa) - l2^2  ;
f3 = (Rp*B3 + P - Ra*A3 - Oa)'*(Rp*B3 + P - Ra*A3 - Oa) - l3^2  ;

df1z = Pz - az + conj(Pz) - conj(az) - (a*sin(conj(beta)))/2 - (conj(a)*sin(beta))/2 + (3^(1/2)*conj(a)*cos(beta)*sin(alpha))/2 + (3^(1/2)*a*cos(conj(beta))*sin(conj(alpha)))/2;
 
 
df1_alpha = (3^(1/2)*a*(cos(conj(gamma))*sin(conj(alpha)) - cos(conj(alpha))*sin(conj(beta))*sin(conj(gamma)))*((conj(a)*sin(gamma))/2 + (3^(1/2)*conj(a)*cos(gamma))/2 - (conj(a)*cos(beta)*cos(gamma))/2 - (3^(1/2)*conj(a)*(cos(alpha)*cos(gamma) + sin(alpha)*sin(beta)*sin(gamma)))/2))/2 - (3^(1/2)*a*(sin(conj(alpha))*sin(conj(gamma)) + cos(conj(alpha))*cos(conj(gamma))*sin(conj(beta)))*((conj(a)*cos(gamma))/2 - (3^(1/2)*conj(a)*sin(gamma))/2 - (conj(a)*cos(beta)*cos(gamma))/2 + (3^(1/2)*conj(a)*(cos(alpha)*sin(gamma) - cos(gamma)*sin(alpha)*sin(beta)))/2))/2 - (3^(1/2)*conj(a)*(sin(alpha)*sin(gamma) + cos(alpha)*cos(gamma)*sin(beta))*((a*cos(conj(gamma)))/2 - (a*cos(conj(beta))*cos(conj(gamma)))/2 + (3^(1/2)*a*(cos(conj(alpha))*sin(conj(gamma)) - cos(conj(gamma))*sin(conj(alpha))*sin(conj(beta))))/2 - (3^(1/2)*a*sin(conj(gamma)))/2))/2 + (3^(1/2)*conj(a)*(cos(gamma)*sin(alpha) - cos(alpha)*sin(beta)*sin(gamma))*((a*sin(conj(gamma)))/2 - (a*cos(conj(beta))*cos(conj(gamma)))/2 - (3^(1/2)*a*(cos(conj(alpha))*cos(conj(gamma)) + sin(conj(alpha))*sin(conj(beta))*sin(conj(gamma))))/2 + (3^(1/2)*a*cos(conj(gamma)))/2))/2 + (3^(1/2)*a*cos(conj(alpha))*cos(conj(beta))*(conj(Pz) - conj(az) - (conj(a)*sin(beta))/2 + (3^(1/2)*conj(a)*cos(beta)*sin(alpha))/2))/2 + (3^(1/2)*conj(a)*cos(alpha)*cos(beta)*(Pz - az - (a*sin(conj(beta)))/2 + (3^(1/2)*a*cos(conj(beta))*sin(conj(alpha)))/2))/2;
 
 
df1_beta = ((conj(a)*cos(gamma)*sin(beta))/2 - (3^(1/2)*conj(a)*cos(beta)*cos(gamma)*sin(alpha))/2)*((a*cos(conj(gamma)))/2 - (a*cos(conj(beta))*cos(conj(gamma)))/2 + (3^(1/2)*a*(cos(conj(alpha))*sin(conj(gamma)) - cos(conj(gamma))*sin(conj(alpha))*sin(conj(beta))))/2 - (3^(1/2)*a*sin(conj(gamma)))/2) + ((conj(a)*cos(gamma)*sin(beta))/2 - (3^(1/2)*conj(a)*cos(beta)*sin(alpha)*sin(gamma))/2)*((a*sin(conj(gamma)))/2 - (a*cos(conj(beta))*cos(conj(gamma)))/2 - (3^(1/2)*a*(cos(conj(alpha))*cos(conj(gamma)) + sin(conj(alpha))*sin(conj(beta))*sin(conj(gamma))))/2 + (3^(1/2)*a*cos(conj(gamma)))/2) - ((a*cos(conj(beta)))/2 + (3^(1/2)*a*sin(conj(alpha))*sin(conj(beta)))/2)*(conj(Pz) - conj(az) - (conj(a)*sin(beta))/2 + (3^(1/2)*conj(a)*cos(beta)*sin(alpha))/2) + ((a*cos(conj(gamma))*sin(conj(beta)))/2 - (3^(1/2)*a*cos(conj(beta))*cos(conj(gamma))*sin(conj(alpha)))/2)*((conj(a)*cos(gamma))/2 - (3^(1/2)*conj(a)*sin(gamma))/2 - (conj(a)*cos(beta)*cos(gamma))/2 + (3^(1/2)*conj(a)*(cos(alpha)*sin(gamma) - cos(gamma)*sin(alpha)*sin(beta)))/2) + ((a*cos(conj(gamma))*sin(conj(beta)))/2 - (3^(1/2)*a*cos(conj(beta))*sin(conj(alpha))*sin(conj(gamma)))/2)*((conj(a)*sin(gamma))/2 + (3^(1/2)*conj(a)*cos(gamma))/2 - (conj(a)*cos(beta)*cos(gamma))/2 - (3^(1/2)*conj(a)*(cos(alpha)*cos(gamma) + sin(alpha)*sin(beta)*sin(gamma)))/2) - ((conj(a)*cos(beta))/2 + (3^(1/2)*conj(a)*sin(alpha)*sin(beta))/2)*(Pz - az - (a*sin(conj(beta)))/2 + (3^(1/2)*a*cos(conj(beta))*sin(conj(alpha)))/2);
 
 
df2z = Pz - az + conj(Pz) - conj(az) + a*sin(conj(beta)) + conj(a)*sin(beta);
 
 
df2_alpha = 0;
 
 
df2_beta = a*cos(conj(beta))*(conj(Pz) - conj(az) + conj(a)*sin(beta)) + conj(a)*cos(beta)*(Pz - az + a*sin(conj(beta))) + a*cos(conj(gamma))*sin(conj(beta))*(conj(a)*cos(gamma) - conj(a)*cos(beta)*cos(gamma)) + conj(a)*cos(gamma)*sin(beta)*(a*cos(conj(gamma)) - a*cos(conj(beta))*cos(conj(gamma))) + a*cos(conj(gamma))*sin(conj(beta))*(conj(a)*sin(gamma) - conj(a)*cos(beta)*cos(gamma)) + conj(a)*cos(gamma)*sin(beta)*(a*sin(conj(gamma)) - a*cos(conj(beta))*cos(conj(gamma)));
 
 
df3z = Pz - az + conj(Pz) - conj(az) - (a*sin(conj(beta)))/2 - (conj(a)*sin(beta))/2 - (3^(1/2)*conj(a)*cos(beta)*sin(alpha))/2 - (3^(1/2)*a*cos(conj(beta))*sin(conj(alpha)))/2;
 
 
df3_alpha = (3^(1/2)*a*(sin(conj(alpha))*sin(conj(gamma)) + cos(conj(alpha))*cos(conj(gamma))*sin(conj(beta)))*((conj(a)*cos(gamma))/2 + (3^(1/2)*conj(a)*sin(gamma))/2 - (conj(a)*cos(beta)*cos(gamma))/2 - (3^(1/2)*conj(a)*(cos(alpha)*sin(gamma) - cos(gamma)*sin(alpha)*sin(beta)))/2))/2 - (3^(1/2)*a*(cos(conj(gamma))*sin(conj(alpha)) - cos(conj(alpha))*sin(conj(beta))*sin(conj(gamma)))*((conj(a)*sin(gamma))/2 - (3^(1/2)*conj(a)*cos(gamma))/2 - (conj(a)*cos(beta)*cos(gamma))/2 + (3^(1/2)*conj(a)*(cos(alpha)*cos(gamma) + sin(alpha)*sin(beta)*sin(gamma)))/2))/2 + (3^(1/2)*conj(a)*(sin(alpha)*sin(gamma) + cos(alpha)*cos(gamma)*sin(beta))*((a*cos(conj(gamma)))/2 - (a*cos(conj(beta))*cos(conj(gamma)))/2 - (3^(1/2)*a*(cos(conj(alpha))*sin(conj(gamma)) - cos(conj(gamma))*sin(conj(alpha))*sin(conj(beta))))/2 + (3^(1/2)*a*sin(conj(gamma)))/2))/2 - (3^(1/2)*conj(a)*(cos(gamma)*sin(alpha) - cos(alpha)*sin(beta)*sin(gamma))*((a*sin(conj(gamma)))/2 - (a*cos(conj(beta))*cos(conj(gamma)))/2 + (3^(1/2)*a*(cos(conj(alpha))*cos(conj(gamma)) + sin(conj(alpha))*sin(conj(beta))*sin(conj(gamma))))/2 - (3^(1/2)*a*cos(conj(gamma)))/2))/2 + (3^(1/2)*a*cos(conj(alpha))*cos(conj(beta))*(conj(az) - conj(Pz) + (conj(a)*sin(beta))/2 + (3^(1/2)*conj(a)*cos(beta)*sin(alpha))/2))/2 + (3^(1/2)*conj(a)*cos(alpha)*cos(beta)*(az - Pz + (a*sin(conj(beta)))/2 + (3^(1/2)*a*cos(conj(beta))*sin(conj(alpha)))/2))/2;
 
 
df3_beta = ((conj(a)*cos(gamma)*sin(beta))/2 + (3^(1/2)*conj(a)*cos(beta)*cos(gamma)*sin(alpha))/2)*((a*cos(conj(gamma)))/2 - (a*cos(conj(beta))*cos(conj(gamma)))/2 - (3^(1/2)*a*(cos(conj(alpha))*sin(conj(gamma)) - cos(conj(gamma))*sin(conj(alpha))*sin(conj(beta))))/2 + (3^(1/2)*a*sin(conj(gamma)))/2) + ((conj(a)*cos(gamma)*sin(beta))/2 + (3^(1/2)*conj(a)*cos(beta)*sin(alpha)*sin(gamma))/2)*((a*sin(conj(gamma)))/2 - (a*cos(conj(beta))*cos(conj(gamma)))/2 + (3^(1/2)*a*(cos(conj(alpha))*cos(conj(gamma)) + sin(conj(alpha))*sin(conj(beta))*sin(conj(gamma))))/2 - (3^(1/2)*a*cos(conj(gamma)))/2) + ((a*cos(conj(beta)))/2 - (3^(1/2)*a*sin(conj(alpha))*sin(conj(beta)))/2)*(conj(az) - conj(Pz) + (conj(a)*sin(beta))/2 + (3^(1/2)*conj(a)*cos(beta)*sin(alpha))/2) + ((a*cos(conj(gamma))*sin(conj(beta)))/2 + (3^(1/2)*a*cos(conj(beta))*cos(conj(gamma))*sin(conj(alpha)))/2)*((conj(a)*cos(gamma))/2 + (3^(1/2)*conj(a)*sin(gamma))/2 - (conj(a)*cos(beta)*cos(gamma))/2 - (3^(1/2)*conj(a)*(cos(alpha)*sin(gamma) - cos(gamma)*sin(alpha)*sin(beta)))/2) + ((a*cos(conj(gamma))*sin(conj(beta)))/2 + (3^(1/2)*a*cos(conj(beta))*sin(conj(alpha))*sin(conj(gamma)))/2)*((conj(a)*sin(gamma))/2 - (3^(1/2)*conj(a)*cos(gamma))/2 - (conj(a)*cos(beta)*cos(gamma))/2 + (3^(1/2)*conj(a)*(cos(alpha)*cos(gamma) + sin(alpha)*sin(beta)*sin(gamma)))/2) + ((conj(a)*cos(beta))/2 - (3^(1/2)*conj(a)*sin(alpha)*sin(beta))/2)*(az - Pz + (a*sin(conj(beta)))/2 + (3^(1/2)*a*cos(conj(beta))*sin(conj(alpha)))/2);

f = [f1 f2 f3]';

df = [df1z df1_alpha df1_beta;
      df2z df2_alpha df2_beta;   
      df3z df3_alpha df3_beta];

  
X = X - (df^(-1))*f;

end
 
X(1) = abs(X(1));
y = X;

end
